simulink model "TL"  (Simulink 6.0)
settings: Solver=ode45  StartTime=0  StopTime=10  RelTol=1e-3
settings Model: Creator=Administrator  LastModifiedBy=John

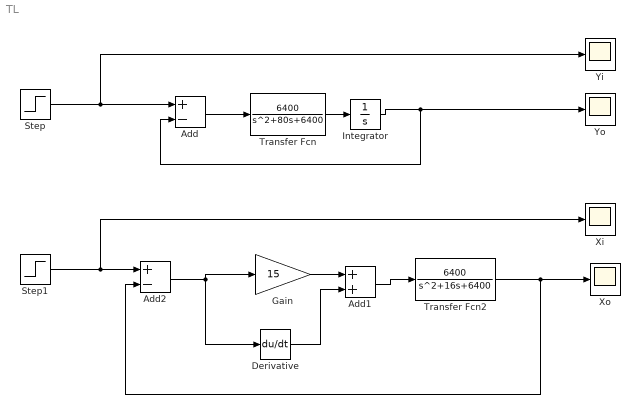
== system TL ==
  Add : Sum  Inputs=+-  OutScaling=2^-10
  Add1 : Sum  OutScaling=2^-10
  Add2 : Sum  Inputs=+-  OutScaling=2^-10
  Derivative : Derivative  LinearizePole=0.02
  Gain : Gain  Gain=15
  Integrator : Integrator
  Step : Step  Time=0.1  SampleTime=0
  Step1 : Step  Time=0.1  SampleTime=0
  Transfer Fcn : TransferFcn  Numerator=[6400]  Denominator=[1 80 6400]
  Transfer Fcn2 : TransferFcn  Numerator=[6400]  Denominator=[1 16 6400]
  Xi : Scope
      settings: TimeRange=15  YMin=0  YMax=200  SaveName=Xi  DataFormat=Array
  Xo : Scope
      settings: SaveName=Xo  DataFormat=Array  MaxDataPoints=210
  Yi : Scope
      settings: TimeRange=20  YMin=0  YMax=160  SaveName=Yi  DataFormat=Array  MaxDataPoints=500
  Yo : Scope
      settings: SaveName=Yo  DataFormat=Array  MaxDataPoints=210
  wires:
  Transfer Fcn/1 -> Integrator/1
  Add/1 -> Transfer Fcn/1
  Integrator/1 -> Add/2, Yo/1
  Step/1 -> Add/1, Yi/1
  Step1/1 -> Add2/1, Xi/1
  Add2/1 -> Gain/1, Derivative/1
  Derivative/1 -> Add1/2
  Gain/1 -> Add1/1
  Add1/1 -> Transfer Fcn2/1
  Transfer Fcn2/1 -> Xo/1, Add2/2
